simulink model "Reverse_Rendulum"  (R2020a)
settings: Solver=VariableStepAuto  StartTime=0.0  StopTime=20  MaxStep=0.01  RelTol=1e-3
libraries: simulink_extras x1, simulink x1
settings Model: EnablePacing=on  Creator=Gleb  LastModifiedBy=Gleb
settings DataIOCC: ReturnWorkspaceOutputs=off

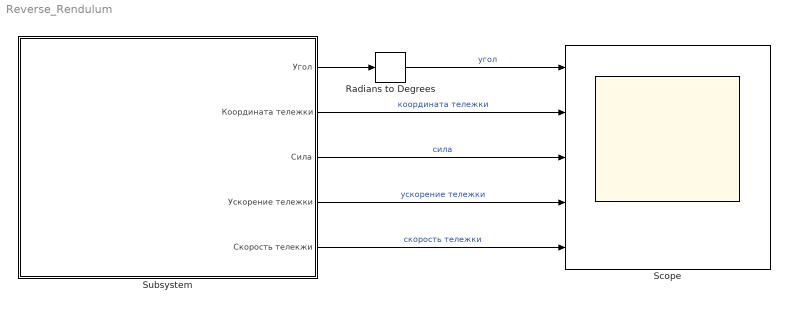
== system Reverse_Rendulum ==
  Radians to Degrees : simulink_extras/Transformations/Radians to Degrees
  Scope : Scope  NumInputPorts=5
  Subsystem : Subsystem  mask{m=1, l=1, b=0.1, Mt=1, g=9.81, startDegree=20}
      mask init:
      | I = m*l^2
  wires:
  Subsystem/1(Угол) -> Radians to Degrees/1
  Subsystem/2(Координата тележки) -> Scope/2  "координата тележки"
  Subsystem/3(Сила) -> Scope/3  "сила"
  Subsystem/4(Ускорение тележки) -> Scope/4  "ускорение тележки"
  Subsystem/5(Скорость телекжи) -> Scope/5  "скорость тележки"
  Radians to Degrees/1 -> Scope/1  "угол"

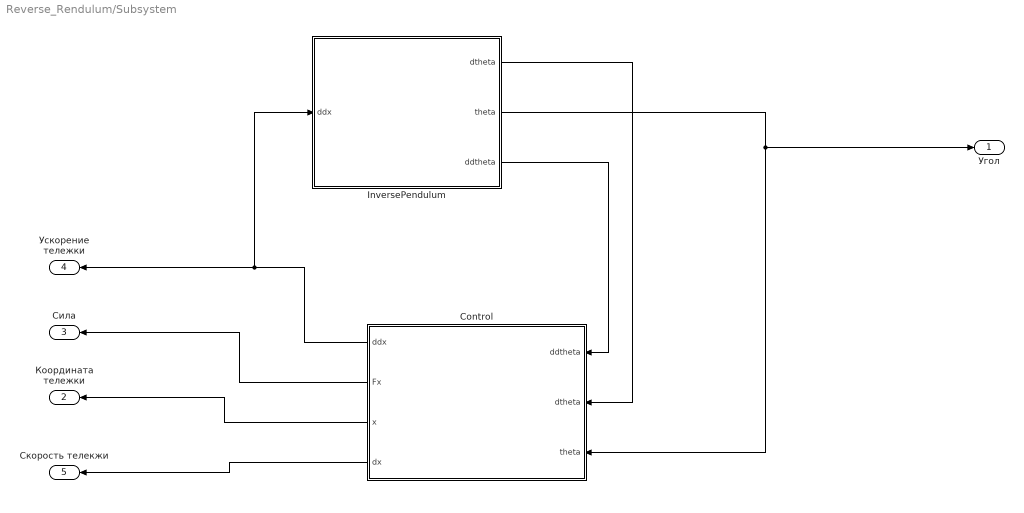
== system Reverse_Rendulum/Subsystem ==
  Control : Subsystem
  InversePendulum : Subsystem
  Угол : Outport
  Координата тележки : Outport  Port=2
  Сила : Outport  Port=3
  Ускорение тележки : Outport  Port=4
  Скорость телекжи : Outport  Port=5
  wires:
  Control/4(dx) -> Скорость телекжи/1
  Control/3(x) -> Координата тележки/1
  Control/2(Fx) -> Сила/1
  Control/1(ddx) -> InversePendulum/1(ddx), Ускорение тележки/1
  InversePendulum/3(ddtheta) -> Control/1(ddtheta)
  InversePendulum/1(dtheta) -> Control/2(dtheta)
  InversePendulum/2(theta) -> Control/3(theta), Угол/1

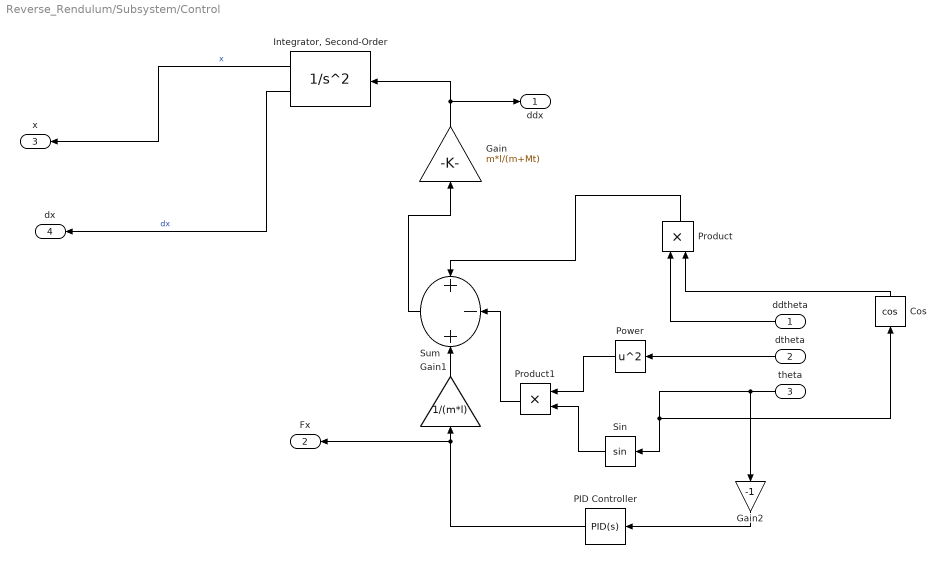
== system Reverse_Rendulum/Subsystem/Control ==
  ddtheta : Inport
  dtheta : Inport  Port=2
  theta : Inport  Port=3
  Cos : Trigonometry  Operator=cos
  Gain : Gain  Gain=m*l/(m+Mt)
  Gain1 : Gain  Gain=1/(m*l)
  Gain2 : Gain  Gain=-1
  "Integrator, Second-Order" : SecondOrderIntegrator
  PID Controller : simulink/Continuous/PID Controller  Controller=PID  Form=Parallel  TimeDomain=Continuous-time  UseExternalTs=off  SampleTime=-1  IntegratorMethod=Forward Euler  FilterMethod=Forward Euler  ControllerParametersSource=internal  P=50  I=50  D=25  UseFilter=on  N=100  TunerSelectOption=Transfer Function Based (PID Tuner App)  InitialConditionSource=internal  InitialConditionForIntegrator=0  InitialConditionForFilter=0  DifferentiatorICPrevScaledInput=0  ExternalReset=none  TrackingMode=off  Kt=1  LimitOutput=off  UpperSaturationLimit=inf  LowerSaturationLimit=-inf  LinearizeAsGain=on  AntiWindupMode=none  Kb=1  POutMin=[]  POutMax=[]  IOutMin=[]  IOutMax=[]  DOutMin=[]  DOutMax=[]  NOutMin=[]  NOutMax=[]  SumOutMin=[]  SumOutMax=[]  SaturationOutMin=[]  SaturationOutMax=[]  PParamMin=[]  PParamMax=[]  IParamMin=[]  IParamMax=[]  DParamMin=[]  DParamMax=[]  NParamMin=[]  NParamMax=[]  KbParamMin=[]  KbParamMax=[]  KtParamMin=[]  KtParamMax=[]  KbOutMin=[]  KbOutMax=[]  KtOutMin=[]  KtOutMax=[]  IntegratorOutMin=[]  IntegratorOutMax=[]  FilterOutMin=[]  FilterOutMax=[]  SumI1OutMin=[]  SumI1OutMax=[]  SumI2OutMin=[]  SumI2OutMax=[]  SumI3OutMin=[]  SumI3OutMax=[]  SumI4OutMin=[]  SumI4OutMax=[]  SumDOutMin=[]  SumDOutMax=[]  DifferentiatorOutMin=[]  DifferentiatorOutMax=[]  FilterDiffOutCoefMin=[]  FilterDiffOutCoefMax=[]  ReciprocalOutMin=[]  ReciprocalOutMax=[]  SumDenOutMin=[]  SumDenOutMax=[]  SumNumOutMin=[]  SumNumOutMax=[]  DivideOutMin=[]  DivideOutMax=[]  UdiffTsProdOutMin=[]  UdiffTsProdOutMax=[]  NTsProdOutMin=[]  NTsProdOutMax=[]  UintegralTsProdOutMin=[]  UintegralTsProdOutMax=[]  UngainTsProdOutMin=[]  UngainTsProdOutMax=[]  IntegratorContinuousStateAttributes=''  IntegratorStateMustResolveToSignalObject=off  IntegratorRTWStateStorageClass=Auto  FilterContinuousStateAttributes=''  FilterStateMustResolveToSignalObject=off  FilterRTWStateStorageClass=Auto  ParallelPVariant=InternalParameters  IdealPVariant=Disabled  IVariant=InternalParameters  DVariant=InternalParameters  IntegratorVariant=Continuous  SatVariant=Disabled  AWVariant=Passthrough  PCopyVariant=Disabled  TRVariant=Disabled  FdbkBlocksVariant=Forward  IdealPFdbkVariant=Disabled  SatFdbkVariant=Disabled  DerivativeFilterVariant=ContFilter  NVariant=InternalParameters  NCopyVariant=Disabled  FilterICVariant=InternalICsFilter  IntegratorICVariant=InternalICs  ExternalResetVariant=Disabled  TRSumVariant=Passthrough  SumFdbkVariant=Disabled  SumVariant=Sum_PID  TsampFilterVariant=InternalTs  TsampNgainVariant=Passthrough  TsampIntegralVariant=Passthrough
  Power : Math  Operator=square  SaturateOnIntegerOverflow=on
  Product : Product
  Product1 : Product
  Sin : Trigonometry
  Sum : Sum  Inputs=+-+
  ddx : Outport
  Fx : Outport  Port=2
  x : Outport  Port=3
  dx : Outport  Port=4
  wires:
  "Integrator, Second-Order"/2 -> dx/1  "dx"
  "Integrator, Second-Order"/1 -> x/1  "x"
  Gain/1 -> "Integrator, Second-Order"/1, ddx/1
  Product/1 -> Sum/1
  Sum/1 -> Gain/1
  dtheta/1 -> Power/1
  Sin/1 -> Product1/2
  Power/1 -> Product1/1
  Product1/1 -> Sum/2
  Cos/1 -> Product/2
  ddtheta/1 -> Product/1
  Gain1/1 -> Sum/3
  theta/1 -> Sin/1, Cos/1, Gain2/1
  Gain2/1 -> PID Controller/1
  PID Controller/1 -> Fx/1, Gain1/1

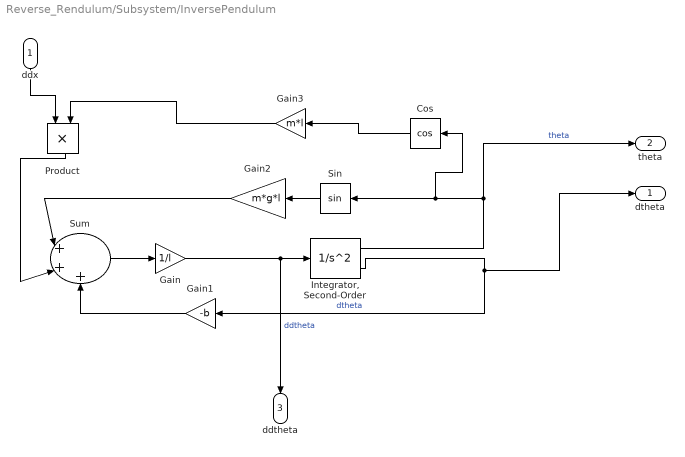
== system Reverse_Rendulum/Subsystem/InversePendulum ==
  ddx : Inport
  Cos : Trigonometry  Operator=cos
  Gain : Gain  Gain=1/l
  Gain1 : Gain  Gain=-b
  Gain2 : Gain  Gain=m*g*l
  Gain3 : Gain  Gain=m*l
  "Integrator, Second-Order" : SecondOrderIntegrator  ICX=deg2rad(startDegree)
  Product : Product
  Sin : Trigonometry
  Sum : Sum  Inputs=|+++
  dtheta : Outport
  theta : Outport  Port=2
  ddtheta : Outport  Port=3
  wires:
  Gain/1 -> "Integrator, Second-Order"/1, ddtheta/1  "ddtheta"
  "Integrator, Second-Order"/1 -> theta/1, Cos/1, Sin/1  "theta"
  "Integrator, Second-Order"/2 -> Gain1/1, dtheta/1  "dtheta"
  Sin/1 -> Gain2/1
  Gain1/1 -> Sum/3
  Gain2/1 -> Sum/1
  Cos/1 -> Gain3/1
  ddx/1 -> Product/1
  Gain3/1 -> Product/2
  Product/1 -> Sum/2
  Sum/1 -> Gain/1
